simulink model "dvss"  (Simulink 3.00)
settings: Solver=ode45  StartTime=0.0  StopTime=10.0  RelTol=1e-3
values from neighbouring files (symbols this model uses):
  A = [-0.417674671349  -0.434751931153  -0.606482859277; -0.595490902619  -0.982300450289  -1.34736267385; -0.149667743824  1.53515226612  -0.433587107399]    [dvss.mat]
  B = [-0.903566942618  0.535397954249; 0.0358796387295  0.552883517424; -0.627531219967  -0.203690479567]    [dvss.mat]
  C = [-2.05432468056  1.59294070377  -1.5804024993; 0.132560731417  1.01841178862  -0.0786619193595]    [dvss.mat]
  D = [-0.681656860002  -1.23435347798; -1.02455305743  0.28880701873]    [dvss.mat]
  ni = 2    [dvss.mat]
  no = 2    [dvss.mat]
  ns = 3    [dvss.mat]
  T = 0.0125    [dvss.mat]
  w = 0    [dvss.mat]
  x0 = 0    [dvss.mat]
libraries: SMXL x10
settings Model: ExtModeTrigMode=normal  ExtModeArmWhenConnect=on  Creator=CAMPA

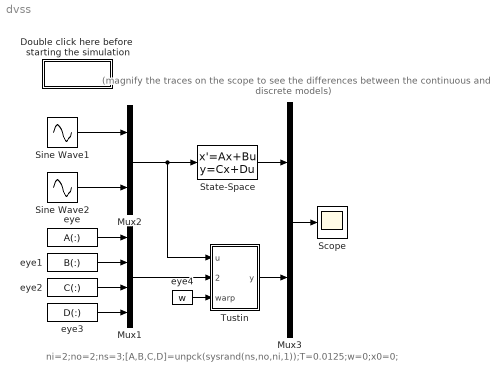
== system dvss ==
  note: ni=2;no=2;ns=3;[A,B,C,D]=unpck(sysrand(ns,no,ni,1));T=0.0125;w=0;x0=0;
  note: (magnify the traces on the scope to see the differences
      | between the continuous and discrete models)
  Double click here before  starting the simulation : Subsystem
      settings: OpenFcn=load dvss
      mask Display: disp('Load Model')
  Mux1 : Mux  Inputs=[ns*ns ns*ni no*ns no*ni]
  Mux2 : Mux  Inputs=2
  Mux3 : Mux  Inputs=2
  Scope : Scope
      settings: TimeRange=10  YMin=-4  YMax=4  SaveToWorkspace=off  SaveName=ScopeData
  Sine Wave1 : Sin  Amplitude=1  Frequency=1.5  Phase=pi/4  SampleTime=0
  Sine Wave2 : Sin  Amplitude=1  Frequency=2  Phase=pi/4  SampleTime=0
  State-Space : StateSpace  A=A  B=B  C=C  D=D  X0=0
  Tustin : Subsystem  mask(Tustin Variable State Space System){ns=ns, no=no, ni=ni, x0=x0, T=T}
      mask prompts: ns "Number of states"; no "Number of Outputs"; ni "Number of Inputs"; x0 "Initial Condition"; T "Sample Time"
      mask help:
      | Simulates a continuous time system A,B,C,D with u as input
      |   and y as output. The four (possibly time varying) matrices are
      |   taken as the second block input and are internally converted
      |   into their discrete time equivalents using a warped bilinear
      |   transform  (warp frequency in rad/s is the 3rd input).
      mask Help:
      | <p>
      |   Simulates a continuous time system A,B,C,D with u as input
      |   and y as output. The four (possibly time varying) matrices are
      |   taken as the second block input and are internally converted
      |   into their discrete time equivalents using a warped bilinear
      |   transform  (warp frequency in rad/s is the 3rd input).
      | </p>
  eye : Constant  Value=A(:)
  eye1 : Constant  Value=B(:)
  eye2 : Constant  Value=C(:)
  eye3 : Constant  Value=D(:)
  eye4 : Constant  Value=w
  wires:
  State-Space/1 -> Mux3/1
  eye4/1 -> Tustin/3(warp)
  eye/1 -> Mux1/1
  eye1/1 -> Mux1/2
  eye2/1 -> Mux1/3
  eye3/1 -> Mux1/4
  Mux1/1 -> Tustin/2(ABCD)
  Tustin/1(y) -> Mux3/2
  Mux3/1 -> Scope/1
  Sine Wave2/1 -> Mux2/2
  Sine Wave1/1 -> Mux2/1
  Mux2/1 -> State-Space/1, Tustin/1(u)

== system dvss/Double click here before  starting the simulation ==

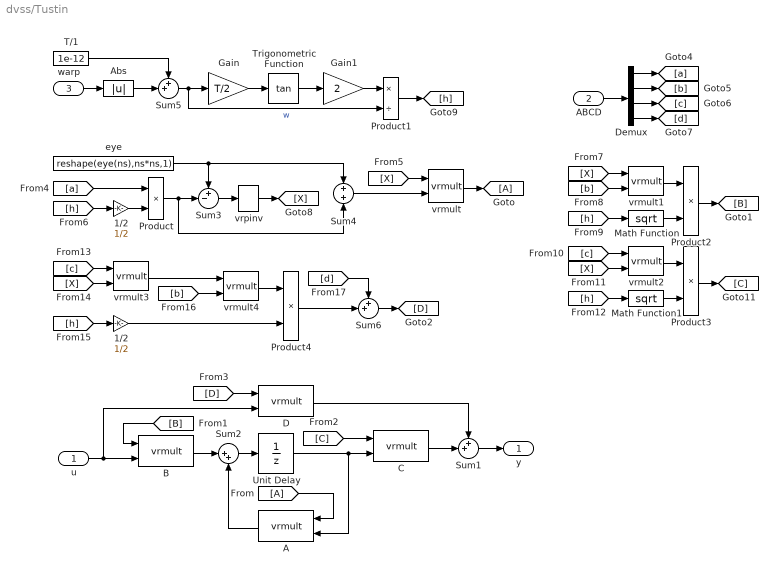
== system dvss/Tustin ==
  u : Inport  Port=1  PortWidth=-1  SampleTime=-1  DataType=auto
      settings: SignalType=auto
  ABCD : Inport  Port=2  PortWidth=-1  SampleTime=-1  DataType=auto
      settings: SignalType=auto
  warp : Inport  Port=3  PortWidth=-1  SampleTime=-1  DataType=auto
      settings: SignalType=auto
  " 1/2 " : Gain  Gain=1/2  SaturateOnIntegerOverflow=on
  1/2 : Gain  Gain=1/2  SaturateOnIntegerOverflow=on
  A : SMXL/Real Matrices/vrmult  Orientation=left  dims=[ns ns 1]
  Abs : Abs
  B : SMXL/Real Matrices/vrmult  dims=[ns ni 1]
  C : SMXL/Real Matrices/vrmult  dims=[no ns 1]
  D : SMXL/Real Matrices/vrmult  dims=[no ni 1]
  Demux : Demux  Outputs=[ns*ns ns*ni no*ns no*ni]
  Gain : Gain  Gain=T/2  SaturateOnIntegerOverflow=on
  Gain1 : Gain  Gain=2  SaturateOnIntegerOverflow=on
  Math Function : Math  Operator=sqrt  OutputSignalType=auto
  Math Function1 : Math  Operator=sqrt  OutputSignalType=auto
  Product{,2..4} (4 alike) : Product  Inputs=2  SaturateOnIntegerOverflow=on
  Product1 : Product  Inputs=*/  SaturateOnIntegerOverflow=on
  Sum1 : Sum  Inputs=++|  SaturateOnIntegerOverflow=on
  Sum2 : Sum  Inputs=|++  SaturateOnIntegerOverflow=on
  Sum3 : Sum  Inputs=+-|  SaturateOnIntegerOverflow=on
  Sum4 : Sum  Inputs=++  SaturateOnIntegerOverflow=on
  Sum5 : Sum  Inputs=++|  SaturateOnIntegerOverflow=on
  Sum6 : Sum  Inputs=++|  SaturateOnIntegerOverflow=on
  T/1 : Constant  Value=1e-12
  Trigonometric Function : Trigonometry  Operator=tan  OutputSignalType=auto
  Unit Delay : UnitDelay  X0=x0  SampleTime=T
  eye : Constant  Value=reshape(eye(ns),ns*ns,1)
  vrmult : SMXL/Real Matrices/vrmult  dims=[ns ns ns]
  vrmult1 : SMXL/Real Matrices/vrmult  dims=[ns ns ni]
  vrmult2 : SMXL/Real Matrices/vrmult  dims=[no ns ns]
  vrmult3 : SMXL/Real Matrices/vrmult  dims=[no ns ns]
  vrmult4 : SMXL/Real Matrices/vrmult  dims=[no ns ni]
  vrpinv : SMXL/Real Matrices/vrpinv  dims=[ns ns]  tol=1
  y : Outport  Port=1
  wires:
  Sum2/1 -> Unit Delay/1
  Sum1/1 -> y/1
  Demux/1 -> [a]
  Demux/2 -> [b]
  Demux/3 -> [c]
  Demux/4 -> [d]
  ABCD/1 -> Demux/1
  eye/1 -> Sum3/1, Sum4/1
  [a] -> Product/1
  [h] -> 1/2/1
  Product/1 -> Sum3/2, Sum4/2
  warp/1 -> Abs/1
  Sum5/1 -> Gain/1, Product1/2  "w"
  Abs/1 -> Sum5/2
  T/1/1 -> Sum5/1
  Gain/1 -> Trigonometric Function/1
  Trigonometric Function/1 -> Gain1/1
  Gain1/1 -> Product1/1
  Product1/1 -> [h]
  1/2/1 -> Product/2
  [h] -> Math Function/1
  Math Function/1 -> Product2/2
  Product2/1 -> [B]
  [h] -> Math Function1/1
  Math Function1/1 -> Product3/2
  Product3/1 -> [C]
  [h] -> " 1/2 "/1
  " 1/2 "/1 -> Product4/2
  Product4/1 -> Sum6/2
  [d] -> Sum6/1
  Sum6/1 -> [D]
  [A] -> A/1
  [B] -> B/1
  B/1 -> Sum2/1
  A/1 -> Sum2/2
  [b] -> vrmult1/2
  [X] -> vrmult/1
  Sum4/1 -> vrmult/2
  [X] -> vrmult1/1
  [c] -> vrmult2/1
  [X] -> vrmult2/2
  vrmult2/1 -> Product3/1
  vrmult1/1 -> Product2/1
  [c] -> vrmult3/1
  [X] -> vrmult3/2
  vrmult3/1 -> vrmult4/1
  vrmult4/1 -> Product4/1
  [b] -> vrmult4/2
  [D] -> D/1
  u/1 -> B/2, D/2
  D/1 -> Sum1/1
  C/1 -> Sum1/2
  [C] -> C/1
  Unit Delay/1 -> A/2, C/2
  Sum3/1 -> vrpinv/1
  vrpinv/1 -> [X]
  vrmult/1 -> [A]
